simulink model "sldemo_lct_lut"  (Simulink 7.6)
settings: Solver=FixedStepDiscrete  StartTime=0.0  StopTime=20  FixedStep=1  RelTol=1e-3
PreLoadFcn:
  | LUT3D = single(reshape([1:4*5*6], [4 5 6]));
  | LUT4D = single(reshape([1:4*5*6*2], [4 5 6 2]));
Description:
  | Lookup Tables
settings Model: Creator=The MathWorks Inc.  ExtModeAutoUpdateStatusClock=off
settings DataIOCC: SaveOutput=off  SaveTime=off  SignalLoggingName=sigsOut
settings OptimizationCC: InlineParams=on  InlineInvariantSignals=on  ZeroExternalMemoryAtStartup=off  ZeroInternalMemoryAtStartup=off  InitFltsAndDblsToZero=on  OptimizeModelRefInitCode=on  LifeSpan=1
settings DebuggingCC: SaveWithParameterizedLinksMsg=none  SignalResolutionControl=TryResolveAllWithWarning  SolverPrmCheckMsg=none  MultiTaskDSMMsg=warning  MultiTaskCondExecSysMsg=none
settings HardwareCC: TargetUnknown=on
settings RTWCC: SystemTargetFile=ert.tlc  GenCodeOnly=on  TemplateMakefile=ert_default_tmf  Description=RTW Embedded Coder (no auto configuration)  GenerateReport=on  ProcessScript=ert_make_rtw_hook  IncludeHyperlinkInReport=on  LaunchReport=on  IncludeERTFirstTime=on
settings CodeAppCC: IgnoreCustomStorageClasses=off
settings ERTTargetCC: TargetFcnLib=ansi_tfl_tmw.mat  MultiwordLength=2048  GenerateSampleERTMain=on  IncludeMdlTerminateFcn=off  SuppressErrorStatus=on  InlinedParameterPlacement=NonHierarchical  ERTSrcFileBannerTemplate=example_banner.tlc  ERTHdrFileBannerTemplate=example_banner.tlc  ERTCustomFileTemplate=example_file_process.tlc  ConvertIfToSwitch=off

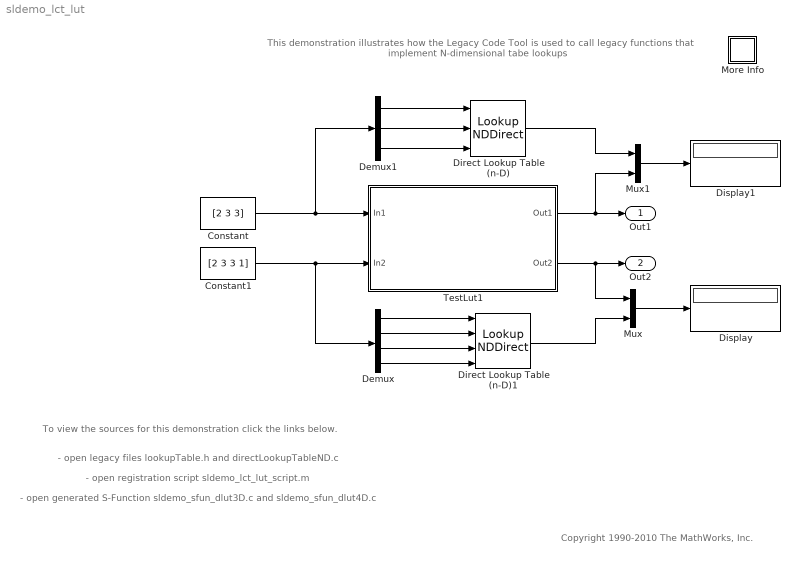
== system sldemo_lct_lut ==
  note: Copyright 1990-2010 The MathWorks, Inc.
  note: This demonstration illustrates how the Legacy Code Tool is used to
      | call legacy functions that implement N-dimensional tabe lookups
  note: - open legacy files lookupTable.h and directLookupTableND.c
  note: To view the sources for this demonstration
      | click the links below.
  note: - open registration script sldemo_lct_lut_script.m
  note: - open generated S-Function sldemo_sfun_dlut3D.c and sldemo_sfun_dlut4D.c
  Constant : Constant  Value=[2 3 3]  OutDataTypeStr=Inherit: Inherit via back propagation  SampleTime=1
  Constant1 : Constant  Value=[2 3 3 1]  OutDataTypeStr=Inherit: Inherit via back propagation  SampleTime=1
  Demux : Demux
  Demux1 : Demux  Outputs=3
  Direct Lookup Table (n-D) : LookupNDDirect  NumberOfTableDimensions=3  Table=LUT3D
  Direct Lookup Table (n-D)1 : LookupNDDirect  NumberOfTableDimensions=4  Table=LUT4D
  Display : Display
  Display1 : Display
  More Info : Subsystem
      settings: OpenFcn=showdemo('sldemo_lct_lut_script')
      mask Display: disp('?')
  Mux : Mux  Inputs=2
  Mux1 : Mux  Inputs=2
  TestLut1 : Subsystem
  Out1 : Outport
  Out2 : Outport  Port=2
  wires:
  TestLut1/1(Out1) -> Out1/1, Mux1/2
  TestLut1/2(Out2) -> Out2/1, Mux/1
  Constant/1 -> TestLut1/1(In1), Demux1/1
  Constant1/1 -> TestLut1/2(In2), Demux/1
  Demux/1 -> Direct Lookup Table (n-D)1/1
  Demux/2 -> Direct Lookup Table (n-D)1/2
  Demux/3 -> Direct Lookup Table (n-D)1/3
  Demux/4 -> Direct Lookup Table (n-D)1/4
  Demux1/1 -> Direct Lookup Table (n-D)/1
  Demux1/2 -> Direct Lookup Table (n-D)/2
  Demux1/3 -> Direct Lookup Table (n-D)/3
  Direct Lookup Table (n-D)1/1 -> Mux/2
  Direct Lookup Table (n-D)/1 -> Mux1/1
  Mux1/1 -> Display1/1
  Mux/1 -> Display/1

== system sldemo_lct_lut/More Info ==

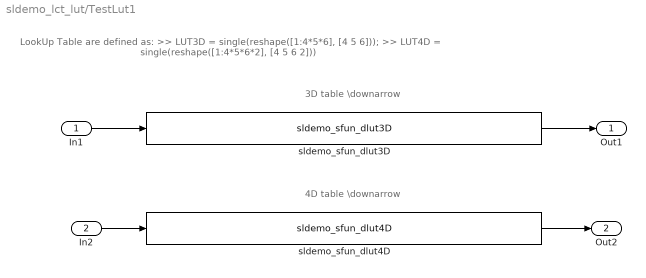
== system sldemo_lct_lut/TestLut1 ==
  note: 3D table
      | \downarrow
  note: 4D table
      | \downarrow
  note: LookUp Table are defined as:
      |       >> LUT3D = single(reshape([1:4*5*6], [4 5 6]));
      |       >> LUT4D = single(reshape([1:4*5*6*2], [4 5 6 2]))
  In1 : Inport
  In2 : Inport  Port=2
  sldemo_sfun_dlut3D : S-Function  FunctionName=sldemo_sfun_dlut3D  Parameters=SParameter1, SParameter2  EnableBusSupport=off  mask(Legacy Function){SFunctionSpec=single y1 = DirectLookupTable3D(single p1[][][], uint32 p2[3], uint32 u1[3]), SParameter1=LUT3D, SParameter2=size(LUT3D), ShowSpec=on}
      mask prompts: SParameter1 "P1:"; SParameter2 "P2:"; ShowSpec "Display function specification"
      mask help:
      | This block allows you to call the legacy functions specified by the following Legacy Code Tool definition:
      | def.SFunctionName = 'sldemo_sfun_dlut3D';
      | def.OutputFcnSpec = 'single y1 = DirectLookupTable3D(single p1[][][], uint32 p2[3], uint32 u1[3])';
      | def.HeaderFiles = {'lookupTable.h'};
      | def.SourceFiles = {'directLookupTableND.c'};
      | def.IncPaths = {'sldemo_lct_src'};
      | def.SrcPaths = {'sldemo_lct_src'};
      mask Help: <p>This block was generated automatically by the Legacy Code Tool. For detailed help on this tool, call<a href="matlab:legacy_code('help')"> legacy_code('help')</a>.</p>
      mask CallbackString:
      | |||if strcmp(get_param(gcbh, 'ShowSpec'), 'on')
      |   set_param(gcbh, 'MaskDisplay', sprintf('fprintf(''%s'');', get_param(gcbh, 'SFunctionSpec')));
      | else
      |   set_param(gcbh, 'MaskDisplay', sprintf('fprintf(''%s'');', get_param(gcbh, 'FunctionName')));
      | end
      mask Display: fprintf('single y1 = DirectLookupTable3D(single p1[][][], uint32 p2[3], uint32 u1[3])');
  sldemo_sfun_dlut4D : S-Function  FunctionName=sldemo_sfun_dlut4D  Parameters=SParameter1, SParameter2  EnableBusSupport=off  mask(Legacy Function){SFunctionSpec=single y1 = DirectLookupTable4D(single p1[][][][], uint32 p2[4], uint32 u1[4]), SParameter1=LUT4D, SParameter2=size(LUT4D), ShowSpec=on}
      mask prompts: SParameter1 "P1:"; SParameter2 "P2:"; ShowSpec "Display function specification"
      mask help:
      | This block allows you to call the legacy functions specified by the following Legacy Code Tool definition:
      | def.SFunctionName = 'sldemo_sfun_dlut4D';
      | def.OutputFcnSpec = 'single y1 = DirectLookupTable4D(single p1[][][][], uint32 p2[4], uint32 u1[4])';
      | def.HeaderFiles = {'lookupTable.h'};
      | def.SourceFiles = {'directLookupTableND.c'};
      | def.IncPaths = {'sldemo_lct_src'};
      | def.SrcPaths = {'sldemo_lct_src'};
      mask Help: <p>This block was generated automatically by the Legacy Code Tool. For detailed help on this tool, call<a href="matlab:legacy_code('help')"> legacy_code('help')</a>.</p>
      mask CallbackString:
      | |||if strcmp(get_param(gcbh, 'ShowSpec'), 'on')
      |   set_param(gcbh, 'MaskDisplay', sprintf('fprintf(''%s'');', get_param(gcbh, 'SFunctionSpec')));
      | else
      |   set_param(gcbh, 'MaskDisplay', sprintf('fprintf(''%s'');', get_param(gcbh, 'FunctionName')));
      | end
      mask Display: fprintf('single y1 = DirectLookupTable4D(single p1[][][][], uint32 p2[4], uint32 u1[4])');
  Out1 : Outport
  Out2 : Outport  Port=2
  wires:
  sldemo_sfun_dlut3D/1 -> Out1/1
  In1/1 -> sldemo_sfun_dlut3D/1
  In2/1 -> sldemo_sfun_dlut4D/1
  sldemo_sfun_dlut4D/1 -> Out2/1
